simulink model "Estimatoare2021b"  (R2022a)
settings: Solver=VariableStepAuto  StartTime=0.0  StopTime=10  RelTol=1e-3
values from neighbouring files (symbols this model uses):
  AEmd = double(eye(12)+Ts*AE)    [EstimareIntrareNecunoscuta.m]    (also in decuplare.m = double(eye(9)+Ts*Adecup))
  Am = double(round(A(1:9,1:9),4))    [ControllerAroundPointOfOperation.m]    (also in InitializeAircraftPlacePolesCalculateN.m = double(round(A(1:9,1:9),2)); newSys.m)
  Amd = (eye(9)+Ts*Am)    [ControlMinimal.m]    (also in ExtendedControl.m; maimultepuncte.m; newSys.m)
  BEmd = double(Ts*BE)    [EstimareIntrareNecunoscuta.m]    (also in decuplare.m = double(Ts*Bdecup))
  Bm = double(round(B(1:9,1:5),4))    [ControllerAroundPointOfOperation.m]    (also in InitializeAircraftPlacePolesCalculateN.m = double(round(B(1:9,1:5),2)); newSys.m)
  Bmd = Ts*Bm    [ControlMinimal.m]    (also in ExtendedControl.m; maimultepuncte.m; newSys.m)
  CEmd = CE    [EstimareIntrareNecunoscuta.m]    (also in decuplare.m)
  Cm = eye(9)    [newSys.m]
  Cmd = Cm    [ControlMinimal.m]    (also in ExtendedControl.m; maimultepuncte.m; newSys.m)
  F = Ft+Rearth2body(0,Theta,Psi)*Fa+R*G    [aircraftSystem.m]    (also in decuplare.m = T*Adecup-K1*CE; proofCerinteLabEstim.m = T*A-K1*C)
  H = H/z    [ControlMinimal.m]    (also in H.m = [1,tan(Theta)*sin(Phi),tan(Theta)*cos(Phi); decuplare.m = E*pinv(CE*E); proofCerinteLabEstim.m = E*pinv(C*E))
  K = K1+K2    [decuplare.m]
  Km = place(Am,Bm,P)    [ControllerAroundPointOfOperation.m]    (also in InitializeAircraftPlacePolesCalculateN.m; newSys.m)
  Kmd = dlqr(Amd,Bmd,Q,R)    [ControlMinimal.m]    (also in ExtendedControl.m; maimultepuncte.m; newSys.m = lqr(Am-Ld*Cmd,Bm,Q,R))
  L = place(Am',Cm',ObsPoles).'    [newSys.m]
  Ld = place(Amd',Cmd',ObsPoles).'    [newSys.m]
  LEd = place(AEmd',CEmd',ObsPoles).'    [EstimareIntrareNecunoscuta.m]
  pointOfEquilibrium = PointOfEquilibrium(operationStates, operatingInputs ,operatingWinds)    [ControllerAroundPointOfOperation.m]    (also in InitializeAircraftPlacePolesCalculateN.m = PointOfEquilibrium([u0;v0;w0;0;0;0;0;Theta0;Psi0;0;0;100].',; TestMergeFinalLoad.m = PointOfEquilibrium(states,inputs,[-1,-1,-1]); extindere_stari_cu_perturbatie.m = PointOfEquilibrium([u0;0;w0;0;0;0;0;Theta0;Psi0;0;0;100].', ; maimultepuncte.m = GetEquilibriumPoint(UW(i),VW(j),WW(k)))
  T = xinputs(1)    [AMatrixAprox.m]    (also in aircraftSystem.m = u(1); decuplare.m = eye(9)-H*CE; proofCerinteLabEstim.m = eye(3)-H*C)
  Ts = 0.1    [ControlMinimal.m]    (also in EstimareIntrareNecunoscuta.m; ExtendedControl.m; KalmanFilterForExtendedLinearSystem.m; LoadmUltiplePoint.m)
  vant = [1,1,1]*0    [EstimareIntrareNecunoscuta.m]    (also in decuplare.m)
undefined symbols (not defined in the file or in its folder): QExt, RExt
libraries: simulink_extras x7
(part 1 of 2)
settings Model: Creator=Bogdan  LastModifiedBy=Bogdan

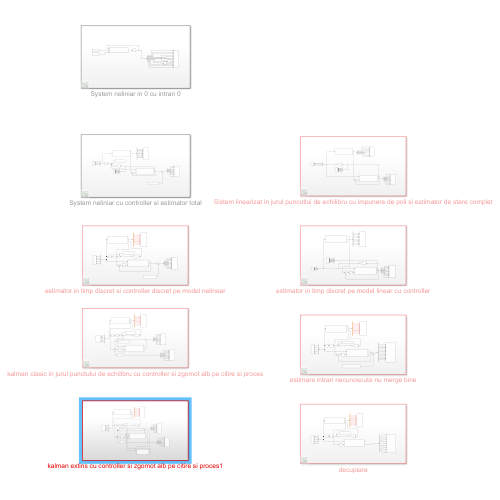
[thumbnail: Simulink's stored preview of the top-level diagram]
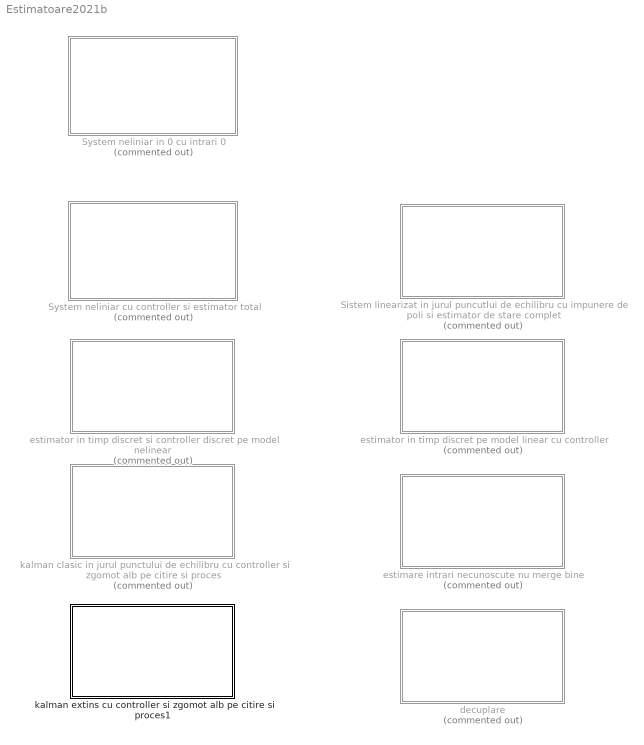
== system Estimatoare2021b ==
  Sistem linearizat in jurul puncutlui de echilibru cu impunere de poli si estimator de stare complet : Subsystem  Description=|  Commented=on
      | Foloseste matricile Am,Bm si Km calculate dupa linearizare in jurul lui 0 cu 
      | %%
      | Am=double(round(A(1:9,1:9),2));
      | Bm=double(round(B(1:9,1:4),2));
      | rank(ctrb(Am,Bm))
      | vpa(eig(Am),2)
      | P=[-.1,-.2,-.3,-.4,-.7,-.8,-1.4,-.15,-7];
      | Km=place(Am,Bm,P)
      | eig(Am-Bm*Km)
  System neliniar cu controller si estimator total : Subsystem  Commented=on
  System neliniar in 0 cu intrari 0 : Subsystem  Commented=on
  decuplare : Subsystem  Description=|  Commented=on
      | Foloseste matricile Am,Bm si Km calculate dupa linearizare in jurul lui 0 cu 
      | %%
      | Am=double(round(A(1:9,1:9),2));
      | Bm=double(round(B(1:9,1:4),2));
      | rank(ctrb(Am,Bm))
      | vpa(eig(Am),2)
      | P=[-.1,-.2,-.3,-.4,-.7,-.8,-1.4,-.15,-7];
      | Km=place(Am,Bm,P)
      | eig(Am-Bm*Km)
  estimare intrari necunoscute nu merge bine : Subsystem  Description=|  Commented=on
      | Foloseste matricile Am,Bm si Km calculate dupa linearizare in jurul lui 0 cu 
      | %%
      | Am=double(round(A(1:9,1:9),2));
      | Bm=double(round(B(1:9,1:4),2));
      | rank(ctrb(Am,Bm))
      | vpa(eig(Am),2)
      | P=[-.1,-.2,-.3,-.4,-.7,-.8,-1.4,-.15,-7];
      | Km=place(Am,Bm,P)
      | eig(Am-Bm*Km)
  estimator in timp discret pe model linear cu controller : Subsystem  Description=|  Commented=on
      | Foloseste matricile Am,Bm si Km calculate dupa linearizare in jurul lui 0 cu 
      | %%
      | Am=double(round(A(1:9,1:9),2));
      | Bm=double(round(B(1:9,1:4),2));
      | rank(ctrb(Am,Bm))
      | vpa(eig(Am),2)
      | P=[-.1,-.2,-.3,-.4,-.7,-.8,-1.4,-.15,-7];
      | Km=place(Am,Bm,P)
      | eig(Am-Bm*Km)
  estimator in timp discret si controller discret pe model nelinear : Subsystem  Description=|  Commented=on
      | Foloseste matricile Am,Bm si Km calculate dupa linearizare in jurul lui 0 cu 
      | %%
      | Am=double(round(A(1:9,1:9),2));
      | Bm=double(round(B(1:9,1:4),2));
      | rank(ctrb(Am,Bm))
      | vpa(eig(Am),2)
      | P=[-.1,-.2,-.3,-.4,-.7,-.8,-1.4,-.15,-7];
      | Km=place(Am,Bm,P)
      | eig(Am-Bm*Km)
  kalman clasic in jurul punctului de echilibru cu controller si zgomot alb pe citire si proces : Subsystem  Description=|  Commented=on
      | Foloseste matricile Am,Bm si Km calculate dupa linearizare in jurul lui 0 cu 
      | %%
      | Am=double(round(A(1:9,1:9),2));
      | Bm=double(round(B(1:9,1:4),2));
      | rank(ctrb(Am,Bm))
      | vpa(eig(Am),2)
      | P=[-.1,-.2,-.3,-.4,-.7,-.8,-1.4,-.15,-7];
      | Km=place(Am,Bm,P)
      | eig(Am-Bm*Km)
  kalman extins cu controller si zgomot alb pe citire si proces1 : Subsystem  Description=|
      | Foloseste matricile Am,Bm si Km calculate dupa linearizare in jurul lui 0 cu 
      | %%
      | Am=double(round(A(1:9,1:9),2));
      | Bm=double(round(B(1:9,1:4),2));
      | rank(ctrb(Am,Bm))
      | vpa(eig(Am),2)
      | P=[-.1,-.2,-.3,-.4,-.7,-.8,-1.4,-.15,-7];
      | Km=place(Am,Bm,P)
      | eig(Am-Bm*Km)

== system Estimatoare2021b/Sistem linearizat in jurul puncutlui de echilibru cu impunere de poli si estimator de stare complet ==
  Controller commands1 : Scope  NumInputPorts=4
  Demux1 : Demux  Outputs=9
  Demux2 : Demux  Outputs=9
  Demux3 : Demux  Outputs=9
  Demux9 : Demux
  Gain1 : Gain  Gain=-Km  Multiplication=Matrix(K*u) (u vector)
  Sum : Sum  Inputs=|+-
  X estim : Scope  NumInputPorts=9
  X real : Scope  NumInputPorts=9
  stari control : Scope  NumInputPorts=9
  system linearizat : Subsystem
  system linearizat1 : Subsystem
  wires:
  Demux9/4 -> Controller commands1/4
  Demux9/2 -> Controller commands1/2
  system linearizat/1(y) -> Sum/1
  Demux9/3 -> Controller commands1/3
  Demux9/1 -> Controller commands1/1
  Demux1/7 -> stari control/7
  Demux1/1 -> stari control/1
  Demux1/8 -> stari control/8
  Demux1/5 -> stari control/5
  Demux1/2 -> stari control/2
  Demux1/3 -> stari control/3
  Demux1/9 -> stari control/9
  Demux1/4 -> stari control/4
  Demux1/6 -> stari control/6
  Demux2/8 -> X real/8
  Demux2/1 -> X real/1
  Demux2/4 -> X real/4
  Demux2/6 -> X real/6
  Demux2/7 -> X real/7
  Demux2/2 -> X real/2
  Demux2/5 -> X real/5
  Demux2/3 -> X real/3
  Demux2/9 -> X real/9
  system linearizat/2(stari) -> Demux2/1
  system linearizat1/1(y_hat) -> Sum/2
  Gain1/1 -> system linearizat1/1(u), system linearizat/1(In1), Demux9/1
  Demux3/5 -> X estim/5
  Demux3/8 -> X estim/8
  Demux3/3 -> X estim/3
  Demux3/2 -> X estim/2
  Demux3/1 -> X estim/1
  Demux3/7 -> X estim/7
  Demux3/4 -> X estim/4
  Demux3/6 -> X estim/6
  Demux3/9 -> X estim/9
  system linearizat1/2(stari) -> Demux3/1
  Sum/1 -> system linearizat1/2(Dy)
  system linearizat1/3(control_states) -> Demux1/1, Gain1/1

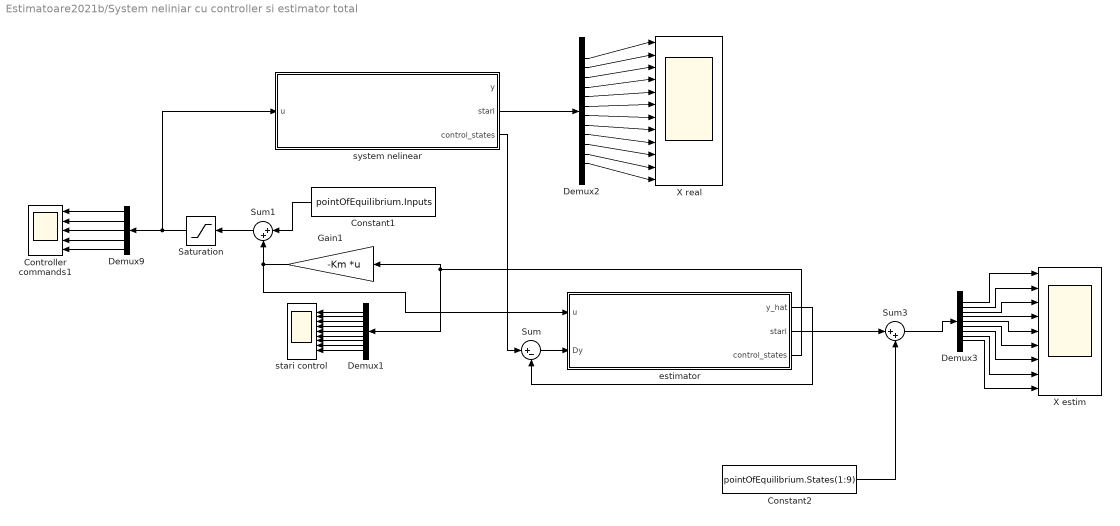
== system Estimatoare2021b/System neliniar cu controller si estimator total ==
  Constant1 : Constant  Value=pointOfEquilibrium.Inputs
  Constant2 : Constant  Value=pointOfEquilibrium.States(1:9)
  Controller commands1 : Scope  NumInputPorts=5
  Demux1 : Demux  Outputs=9
  Demux2 : Demux  Outputs=12
  Demux3 : Demux  Outputs=9
  Demux9 : Demux  Outputs=5
  Gain1 : Gain  Gain=-Km  Multiplication=Matrix(K*u) (u vector)
  Saturation : Saturate  UpperLimit=[10,pi/6,pi/6,pi/6,pi/6]  LowerLimit=[0,-pi/6,-pi/6,-pi/6,-pi/6]
  Sum : Sum  Inputs=|+-
  Sum1 : Sum  Inputs=|++
  Sum3 : Sum  Inputs=|++
  X estim : Scope  NumInputPorts=9
  X real : Scope  NumInputPorts=12
  estimator : Subsystem
  stari control : Scope  NumInputPorts=9
  system nelinear : Subsystem
  wires:
  estimator/1(y_hat) -> Sum/2
  Demux1/8 -> stari control/8
  Demux3/6 -> X estim/6
  system nelinear/2(stari) -> Demux2/1
  Demux3/9 -> X estim/9
  Sum/1 -> estimator/2(Dy)
  Demux1/4 -> stari control/4
  Demux1/3 -> stari control/3
  Demux2/5 -> X real/5
  Demux3/4 -> X estim/4
  Demux2/6 -> X real/6
  Demux2/2 -> X real/2
  Demux3/8 -> X estim/8
  Demux2/9 -> X real/9
  Demux2/8 -> X real/8
  Demux2/3 -> X real/3
  Demux3/2 -> X estim/2
  Demux2/1 -> X real/1
  Demux2/4 -> X real/4
  Demux2/7 -> X real/7
  Demux3/1 -> X estim/1
  Demux3/7 -> X estim/7
  Demux9/1 -> Controller commands1/1
  Demux1/9 -> stari control/9
  Demux1/6 -> stari control/6
  Demux9/3 -> Controller commands1/3
  Demux9/4 -> Controller commands1/4
  Demux1/7 -> stari control/7
  Demux1/2 -> stari control/2
  Demux3/3 -> X estim/3
  Demux1/1 -> stari control/1
  Demux9/2 -> Controller commands1/2
  Demux1/5 -> stari control/5
  Demux3/5 -> X estim/5
  Saturation/1 -> system nelinear/1(u), Demux9/1
  Constant1/1 -> Sum1/1
  Sum1/1 -> Saturation/1
  Gain1/1 -> estimator/1(u), Sum1/2
  estimator/2(stari) -> Sum3/1
  Sum3/1 -> Demux3/1
  Demux2/10 -> X real/10
  Demux2/11 -> X real/11
  Demux2/12 -> X real/12
  Constant2/1 -> Sum3/2
  estimator/3(control_states) -> Gain1/1, Demux1/1
  Demux9/5 -> Controller commands1/5
  system nelinear/3(control_states) -> Sum/1

== system Estimatoare2021b/System neliniar in 0 cu intrari 0 ==
  Constant : Constant  Value=zeros(5,1)
  Constant1 : Constant  Value=zeros(3,1)
  Demux : Demux  Outputs=12
  Integrator : Integrator  InitialCondition=zeros(12,1)
  MATLAB Function : MATLAB Function  TreatAsAtomicUnit=on
  Radians to Degrees : simulink_extras/Transformations/Radians to Degrees
  Radians to Degrees1 : simulink_extras/Transformations/Radians to Degrees
  Radians to Degrees2 : simulink_extras/Transformations/Radians to Degrees
  system states : Scope  NumInputPorts=12
  wires:
  Demux/2 -> system states/2  "v"
  Radians to Degrees2/1 -> system states/9  "Psi"
  Demux/12 -> system states/12  "pozition z in vehicle carried NED"
  MATLAB Function/1(dxdt) -> Integrator/1
  Radians to Degrees/1 -> system states/7  "Phi"
  Demux/10 -> system states/10  "Pozition X in vehicle carried NED"
  Constant/1 -> MATLAB Function/2(u)
  Demux/9 -> Radians to Degrees2/1
  Constant1/1 -> MATLAB Function/3(d)
  Demux/4 -> system states/4  "p"
  Radians to Degrees1/1 -> system states/8  "Theta"
  Demux/3 -> system states/3  "w"
  Integrator/1 -> MATLAB Function/1(x), Demux/1
  Demux/1 -> system states/1  "u"
  Demux/6 -> system states/6  "r"
  Demux/7 -> Radians to Degrees/1
  Demux/8 -> Radians to Degrees1/1
  Demux/11 -> system states/11  "pozition y in vehicle carried NED"
  Demux/5 -> system states/5  "q"

== system Estimatoare2021b/decuplare ==
  Constant1 : Constant  Value=pointOfEquilibrium.Inputs
  Demux : Demux  Outputs=5
  Demux2 : Demux  Outputs=12
  Demux3 : Demux  Outputs=9
  Gain2 : Gain  Gain=-Kmd  Multiplication=Matrix(K*u) (u vector)
  Saturation : Saturate  UpperLimit=[10,pi/6,pi/6,pi/6,pi/6]  LowerLimit=[0,-pi/6,-pi/6,-pi/6,-pi/6]
  Scope : Scope  NumInputPorts=5
  Sum2 : Sum  Inputs=++|
  X estim : Scope  NumInputPorts=9
  X real : Scope  NumInputPorts=12
  Zero-Order Hold : ZeroOrderHold  SampleTime=-1
  Zero-Order Hold1 : ZeroOrderHold  SampleTime=-1
  system linearizat1 : Subsystem
  system nelinear : Subsystem
  wires:
  system nelinear/2(stari) -> Demux2/1
  Demux3/5 -> X estim/5
  Demux3/8 -> X estim/8
  Demux3/3 -> X estim/3
  Demux3/2 -> X estim/2
  Demux3/1 -> X estim/1
  Demux3/7 -> X estim/7
  Demux3/4 -> X estim/4
  Demux3/6 -> X estim/6
  Demux3/9 -> X estim/9
  Demux2/11 -> X real/11
  Demux2/10 -> X real/10
  Demux2/12 -> X real/12
  Demux2/1 -> X real/1
  Demux2/7 -> X real/7
  Demux2/3 -> X real/3
  Demux2/8 -> X real/8
  Demux2/9 -> X real/9
  Demux2/4 -> X real/4
  Demux2/6 -> X real/6
  Demux2/5 -> X real/5
  Demux2/2 -> X real/2
  Gain2/1 -> Sum2/2
  Saturation/1 -> system nelinear/1(u), Demux/1, system linearizat1/1(u)
  Demux/1 -> Scope/1
  Demux/2 -> Scope/2
  Demux/3 -> Scope/3
  Demux/4 -> Scope/4
  Demux/5 -> Scope/5
  Constant1/1 -> Sum2/1
  system nelinear/3(control_states) -> Gain2/1
  system nelinear/1(y) -> Zero-Order Hold/1
  Zero-Order Hold/1 -> system linearizat1/2(Dy)
  Zero-Order Hold1/1 -> Saturation/1
  Sum2/1 -> Zero-Order Hold1/1
  system linearizat1/2(control_states) -> Demux3/1

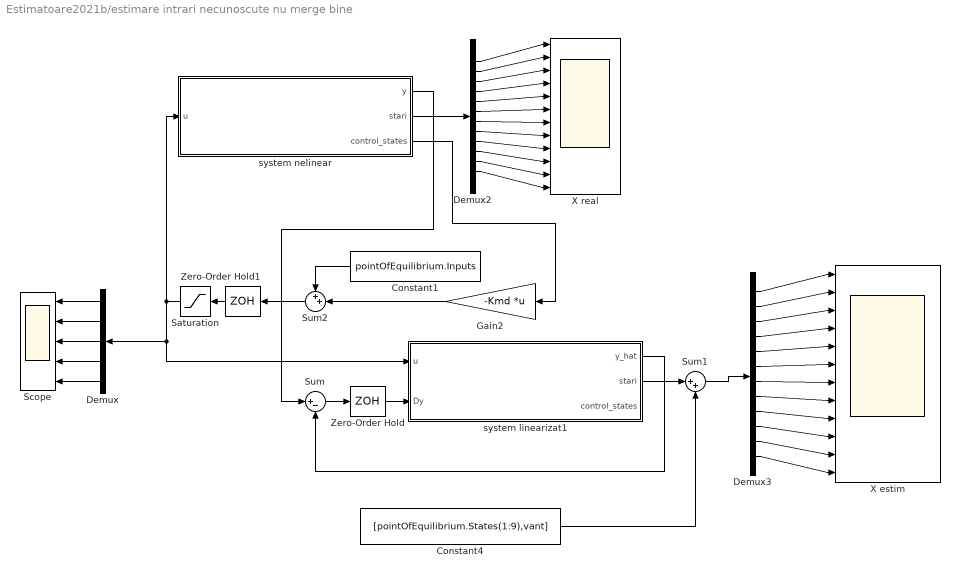
== system Estimatoare2021b/estimare intrari necunoscute nu merge bine ==
  Constant1 : Constant  Value=pointOfEquilibrium.Inputs
  Constant4 : Constant  Value=[pointOfEquilibrium.States(1:9),vant]
  Demux : Demux  Outputs=5
  Demux2 : Demux  Outputs=12
  Demux3 : Demux  Outputs=12
  Gain2 : Gain  Gain=-Kmd  Multiplication=Matrix(K*u) (u vector)
  Saturation : Saturate  UpperLimit=[10,pi/6,pi/6,pi/6,pi/6]  LowerLimit=[0,-pi/6,-pi/6,-pi/6,-pi/6]
  Scope : Scope  NumInputPorts=5
  Sum : Sum  Inputs=|+-
  Sum1 : Sum  Inputs=|++
  Sum2 : Sum  Inputs=++|
  X estim : Scope  NumInputPorts=12
  X real : Scope  NumInputPorts=12
  Zero-Order Hold : ZeroOrderHold  SampleTime=-1
  Zero-Order Hold1 : ZeroOrderHold  SampleTime=-1
  system linearizat1 : Subsystem
  system nelinear : Subsystem
  wires:
  system nelinear/2(stari) -> Demux2/1
  system linearizat1/1(y_hat) -> Sum/2
  Demux3/5 -> X estim/5
  Demux3/8 -> X estim/8
  Demux3/3 -> X estim/3
  Demux3/2 -> X estim/2
  Demux3/1 -> X estim/1
  Demux3/7 -> X estim/7
  Demux3/4 -> X estim/4
  Demux3/6 -> X estim/6
  Demux3/9 -> X estim/9
  Demux2/11 -> X real/11
  Demux2/10 -> X real/10
  Demux2/12 -> X real/12
  Demux2/1 -> X real/1
  Demux2/7 -> X real/7
  Demux2/3 -> X real/3
  Demux2/8 -> X real/8
  Demux2/9 -> X real/9
  Demux2/4 -> X real/4
  Demux2/6 -> X real/6
  Demux2/5 -> X real/5
  Demux2/2 -> X real/2
  Sum1/1 -> Demux3/1
  system linearizat1/2(stari) -> Sum1/1
  Constant4/1 -> Sum1/2
  system nelinear/1(y) -> Sum/1
  Gain2/1 -> Sum2/2
  Saturation/1 -> system nelinear/1(u), Demux/1, system linearizat1/1(u)
  Demux/1 -> Scope/1
  Demux/2 -> Scope/2
  Demux/3 -> Scope/3
  Demux/4 -> Scope/4
  Demux/5 -> Scope/5
  Constant1/1 -> Sum2/1
  Sum/1 -> Zero-Order Hold/1
  Zero-Order Hold/1 -> system linearizat1/2(Dy)
  Zero-Order Hold1/1 -> Saturation/1
  Sum2/1 -> Zero-Order Hold1/1
  Demux3/10 -> X estim/10
  Demux3/11 -> X estim/11
  Demux3/12 -> X estim/12
  system nelinear/3(control_states) -> Gain2/1

== system Estimatoare2021b/estimator in timp discret pe model linear cu controller ==
  Demux : Demux  Outputs=5
  Demux1 : Demux  Outputs=9
  Demux2 : Demux  Outputs=9
  Demux3 : Demux  Outputs=9
  Gain2 : Gain  Gain=-Kmd  Multiplication=Matrix(K*u) (u vector)
  Scope : Scope  NumInputPorts=5
  Sum : Sum  Inputs=|+-
  X estim : Scope  NumInputPorts=9
  X real : Scope  NumInputPorts=9
  Zero-Order Hold2 : ZeroOrderHold  SampleTime=Ts
  stari control : Scope  NumInputPorts=9
  system linearizat : Subsystem
  system linearizat1 : Subsystem
  wires:
  Demux1/7 -> stari control/7
  Demux1/1 -> stari control/1
  Demux1/8 -> stari control/8
  Demux1/5 -> stari control/5
  Demux1/2 -> stari control/2
  Demux1/3 -> stari control/3
  Demux1/9 -> stari control/9
  Demux1/4 -> stari control/4
  Demux1/6 -> stari control/6
  system linearizat/2(stari) -> Demux2/1
  system linearizat1/1(y_hat) -> Sum/2
  Demux3/5 -> X estim/5
  Demux3/8 -> X estim/8
  Demux3/3 -> X estim/3
  Demux3/2 -> X estim/2
  Demux3/1 -> X estim/1
  Demux3/7 -> X estim/7
  Demux3/4 -> X estim/4
  Demux3/6 -> X estim/6
  Demux3/9 -> X estim/9
  system linearizat1/2(stari) -> Demux3/1
  system linearizat/1(y) -> Sum/1
  system linearizat1/3(control_states) -> Gain2/1, Demux1/1
  Gain2/1 -> Demux/1, system linearizat/1(In1), system linearizat1/1(u)
  Zero-Order Hold2/1 -> system linearizat1/2(Dy)
  Sum/1 -> Zero-Order Hold2/1
  Demux2/1 -> X real/1
  Demux2/7 -> X real/7
  Demux2/3 -> X real/3
  Demux2/8 -> X real/8
  Demux2/9 -> X real/9
  Demux2/4 -> X real/4
  Demux2/6 -> X real/6
  Demux2/5 -> X real/5
  Demux2/2 -> X real/2
  Demux/1 -> Scope/1
  Demux/2 -> Scope/2
  Demux/3 -> Scope/3
  Demux/4 -> Scope/4
  Demux/5 -> Scope/5

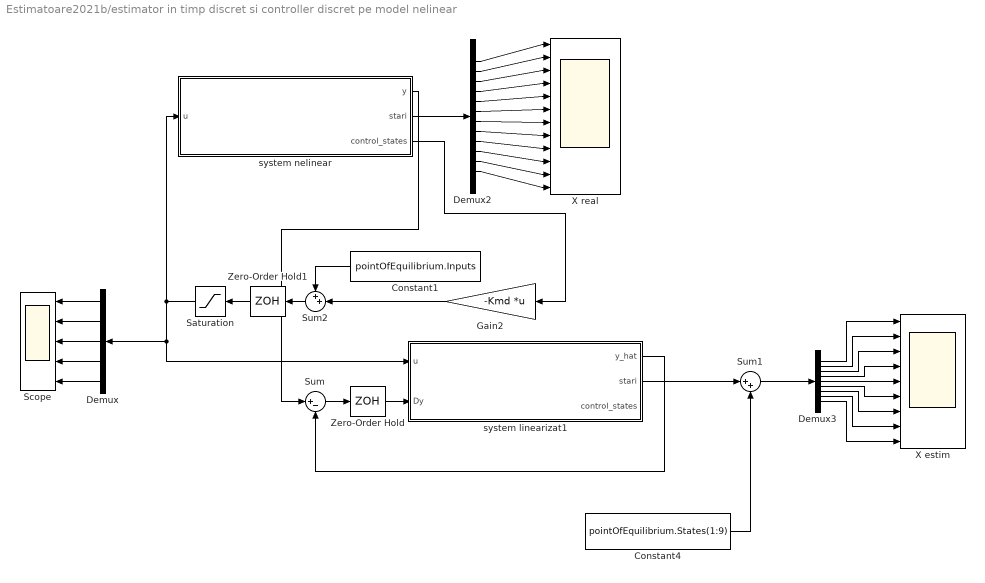
== system Estimatoare2021b/estimator in timp discret si controller discret pe model nelinear ==
  Constant1 : Constant  Value=pointOfEquilibrium.Inputs
  Constant4 : Constant  Value=pointOfEquilibrium.States(1:9)
  Demux : Demux  Outputs=5
  Demux2 : Demux  Outputs=12
  Demux3 : Demux  Outputs=9
  Gain2 : Gain  Gain=-Kmd  Multiplication=Matrix(K*u) (u vector)
  Saturation : Saturate  UpperLimit=[10,pi/6,pi/6,pi/6,pi/6]  LowerLimit=[0,-pi/6,-pi/6,-pi/6,-pi/6]
  Scope : Scope  NumInputPorts=5
  Sum : Sum  Inputs=|+-
  Sum1 : Sum  Inputs=|++
  Sum2 : Sum  Inputs=++|
  X estim : Scope  NumInputPorts=9
  X real : Scope  NumInputPorts=12
  Zero-Order Hold : ZeroOrderHold  SampleTime=-1
  Zero-Order Hold1 : ZeroOrderHold  SampleTime=-1
  system linearizat1 : Subsystem
  system nelinear : Subsystem
  wires:
  system nelinear/2(stari) -> Demux2/1
  system linearizat1/1(y_hat) -> Sum/2
  Demux3/5 -> X estim/5
  Demux3/8 -> X estim/8
  Demux3/3 -> X estim/3
  Demux3/2 -> X estim/2
  Demux3/1 -> X estim/1
  Demux3/7 -> X estim/7
  Demux3/4 -> X estim/4
  Demux3/6 -> X estim/6
  Demux3/9 -> X estim/9
  Demux2/11 -> X real/11
  Demux2/10 -> X real/10
  Demux2/12 -> X real/12
  Demux2/1 -> X real/1
  Demux2/7 -> X real/7
  Demux2/3 -> X real/3
  Demux2/8 -> X real/8
  Demux2/9 -> X real/9
  Demux2/4 -> X real/4
  Demux2/6 -> X real/6
  Demux2/5 -> X real/5
  Demux2/2 -> X real/2
  Sum1/1 -> Demux3/1
  system linearizat1/2(stari) -> Sum1/1
  Constant4/1 -> Sum1/2
  system nelinear/1(y) -> Sum/1
  Gain2/1 -> Sum2/2
  Saturation/1 -> system nelinear/1(u), Demux/1, system linearizat1/1(u)
  Demux/1 -> Scope/1
  Demux/2 -> Scope/2
  Demux/3 -> Scope/3
  Demux/4 -> Scope/4
  Demux/5 -> Scope/5
  Constant1/1 -> Sum2/1
  system nelinear/3(control_states) -> Gain2/1
  Sum/1 -> Zero-Order Hold/1
  Zero-Order Hold/1 -> system linearizat1/2(Dy)
  Zero-Order Hold1/1 -> Saturation/1
  Sum2/1 -> Zero-Order Hold1/1

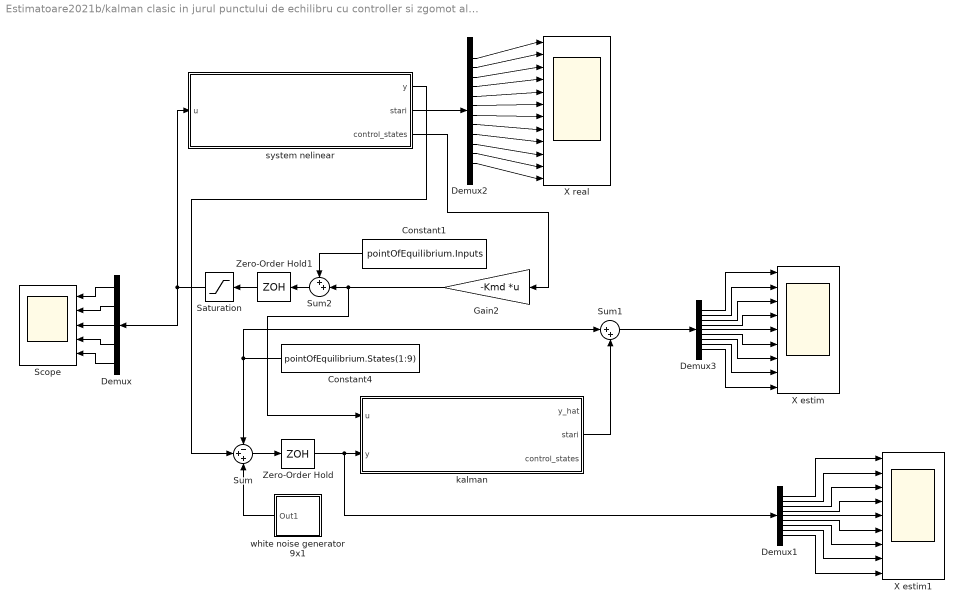
== system Estimatoare2021b/kalman clasic in jurul punctului de echilibru cu controller si zgomot alb pe citire si proces ==
  Constant1 : Constant  Value=pointOfEquilibrium.Inputs
  Constant4 : Constant  Value=pointOfEquilibrium.States(1:9)
  Demux : Demux  Outputs=5
  Demux1 : Demux  Outputs=9
  Demux2 : Demux  Outputs=12
  Demux3 : Demux  Outputs=9
  Gain2 : Gain  Gain=-Kmd  Multiplication=Matrix(K*u) (u vector)
  Saturation : Saturate  UpperLimit=[10,pi/6,pi/6,pi/6,pi/6]  LowerLimit=[0,-pi/6,-pi/6,-pi/6,-pi/6]
  Scope : Scope  NumInputPorts=5
  Sum : Sum  Inputs=-++
  Sum1 : Sum  Inputs=|++
  Sum2 : Sum  Inputs=++|
  X estim : Scope  NumInputPorts=9
  X estim1 : Scope  NumInputPorts=9
  X real : Scope  NumInputPorts=12
  Zero-Order Hold : ZeroOrderHold  SampleTime=-1
  Zero-Order Hold1 : ZeroOrderHold  SampleTime=-1
  kalman : Subsystem
  system nelinear : Subsystem
  white noise generator 9x1 : Subsystem
  wires:
  system nelinear/2(stari) -> Demux2/1
  Demux3/5 -> X estim/5
  Demux3/8 -> X estim/8
  Demux3/3 -> X estim/3
  Demux3/2 -> X estim/2
  Demux3/1 -> X estim/1
  Demux3/7 -> X estim/7
  Demux3/4 -> X estim/4
  Demux3/6 -> X estim/6
  Demux3/9 -> X estim/9
  Demux2/11 -> X real/11
  Demux2/10 -> X real/10
  Demux2/12 -> X real/12
  Demux2/1 -> X real/1
  Demux2/7 -> X real/7
  Demux2/3 -> X real/3
  Demux2/8 -> X real/8
  Demux2/9 -> X real/9
  Demux2/4 -> X real/4
  Demux2/6 -> X real/6
  Demux2/5 -> X real/5
  Demux2/2 -> X real/2
  Gain2/1 -> kalman/1(u), Sum2/2
  Saturation/1 -> system nelinear/1(u), Demux/1
  Demux/1 -> Scope/1
  Demux/2 -> Scope/2
  Demux/3 -> Scope/3
  Demux/4 -> Scope/4
  Demux/5 -> Scope/5
  Constant1/1 -> Sum2/1
  Zero-Order Hold/1 -> Demux1/1, kalman/2(y)
  Zero-Order Hold1/1 -> Saturation/1
  Sum2/1 -> Zero-Order Hold1/1
  Sum/1 -> Zero-Order Hold/1
  Demux1/4 -> X estim1/4
  Demux1/8 -> X estim1/8
  Demux1/7 -> X estim1/7
  Demux1/9 -> X estim1/9
  Demux1/1 -> X estim1/1
  Demux1/6 -> X estim1/6
  Demux1/3 -> X estim1/3
  Demux1/2 -> X estim1/2
  Demux1/5 -> X estim1/5
  white noise generator 9x1/1(Out1) -> Sum/3
  Constant4/1 -> Sum1/1, Sum/1
  system nelinear/1(y) -> Sum/2
  kalman/2(stari) -> Sum1/2
  Sum1/1 -> Demux3/1
  system nelinear/3(control_states) -> Gain2/1

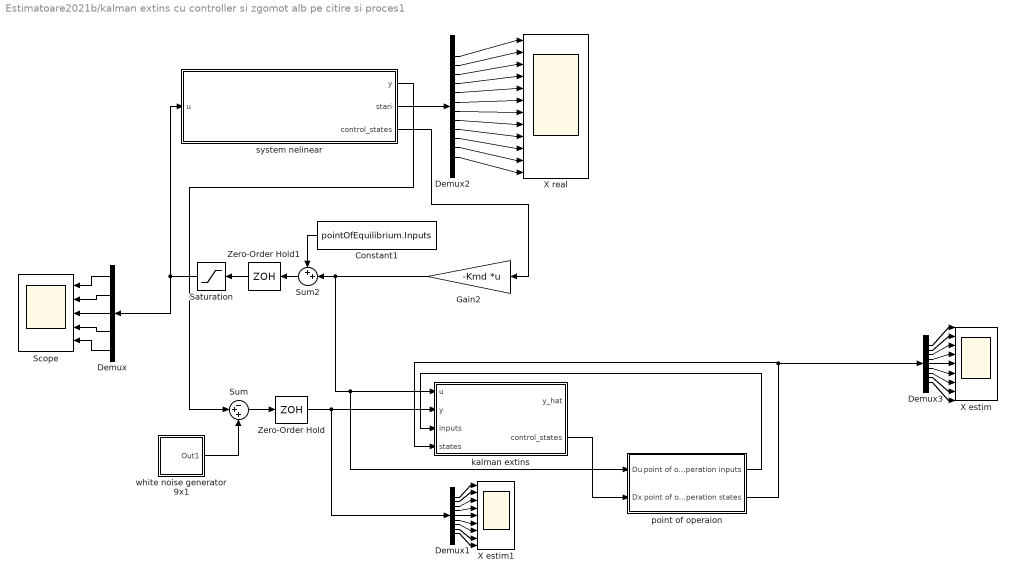
== system Estimatoare2021b/kalman extins cu controller si zgomot alb pe citire si proces1 ==
  Constant1 : Constant  Value=pointOfEquilibrium.Inputs
  Demux : Demux  Outputs=5
  Demux1 : Demux  Outputs=9
  Demux2 : Demux  Outputs=12
  Demux3 : Demux  Outputs=9
  Gain2 : Gain  Gain=-Kmd  Multiplication=Matrix(K*u) (u vector)
  Saturation : Saturate  UpperLimit=[10,pi/6,pi/6,pi/6,pi/6]  LowerLimit=[0,-pi/6,-pi/6,-pi/6,-pi/6]
  Scope : Scope  NumInputPorts=5
  Sum : Sum  Inputs=-++
  Sum2 : Sum  Inputs=++|
  X estim : Scope  NumInputPorts=9
  X estim1 : Scope  NumInputPorts=9
  X real : Scope  NumInputPorts=12
  Zero-Order Hold : ZeroOrderHold  SampleTime=-1
  Zero-Order Hold1 : ZeroOrderHold  SampleTime=-1
  kalman extins : Subsystem
  point of operaion : Subsystem
  system nelinear : Subsystem
  white noise generator 9x1 : Subsystem
  wires:
  system nelinear/2(stari) -> Demux2/1
  Demux3/5 -> X estim/5
  Demux3/8 -> X estim/8
  Demux3/3 -> X estim/3
  Demux3/2 -> X estim/2
  Demux3/1 -> X estim/1
  Demux3/7 -> X estim/7
  Demux3/4 -> X estim/4
  Demux3/6 -> X estim/6
  Demux3/9 -> X estim/9
  Demux2/11 -> X real/11
  Demux2/10 -> X real/10
  Demux2/12 -> X real/12
  Demux2/1 -> X real/1
  Demux2/7 -> X real/7
  Demux2/3 -> X real/3
  Demux2/8 -> X real/8
  Demux2/9 -> X real/9
  Demux2/4 -> X real/4
  Demux2/6 -> X real/6
  Demux2/5 -> X real/5
  Demux2/2 -> X real/2
  Gain2/1 -> point of operaion/1(Du), kalman extins/1(u), Sum2/2
  Saturation/1 -> system nelinear/1(u), Demux/1
  Demux/1 -> Scope/1
  Demux/2 -> Scope/2
  Demux/3 -> Scope/3
  Demux/4 -> Scope/4
  Demux/5 -> Scope/5
  Zero-Order Hold/1 -> Demux1/1, kalman extins/2(y)
  Zero-Order Hold1/1 -> Saturation/1
  Sum2/1 -> Zero-Order Hold1/1
  Sum/1 -> Zero-Order Hold/1
  Demux1/4 -> X estim1/4
  Demux1/8 -> X estim1/8
  Demux1/7 -> X estim1/7
  Demux1/9 -> X estim1/9
  Demux1/1 -> X estim1/1
  Demux1/6 -> X estim1/6
  Demux1/3 -> X estim1/3
  Demux1/2 -> X estim1/2
  Demux1/5 -> X estim1/5
  white noise generator 9x1/1(Out1) -> Sum/3
  system nelinear/1(y) -> Sum/2
  system nelinear/3(control_states) -> Gain2/1
  kalman extins/2(control_states) -> point of operaion/2(Dx)
  Constant1/1 -> Sum2/1
  point of operaion/2(point of operation states) -> Demux3/1, kalman extins/4(states)
  point of operaion/1(point of operation inputs) -> kalman extins/3(inputs)

== system Estimatoare2021b/Sistem linearizat in jurul puncutlui de echilibru cu impunere de poli si estimator de stare complet/system linearizat ==
  In1 : Inport
  Constant1 : Constant  Value=Am
  Constant2 : Constant  Value=Bm
  Constant4 : Constant  Value=pointOfEquilibrium.States(1:9)
  Demux : Demux  Outputs=9
  Gain : Gain  Gain=Cm  Multiplication=Matrix(K*u) (u vector)
  Integrator : Integrator  InitialCondition=pointOfEquilibrium.States(1:9)
  Mux : Mux  Inputs=9
  Product : Product  Multiplication=Matrix(*)
  Product1 : Product  Multiplication=Matrix(*)
  Sum : Sum  Inputs=+++
  Sum1 : Sum  Inputs=+-
  y : Outport
  stari : Outport  Port=2
  control_states : Outport  Port=3
  wires:
  Constant2/1 -> Product1/1
  Integrator/1 -> Sum1/1
  Constant1/1 -> Product/1
  In1/1 -> Product1/2
  Constant4/1 -> Sum1/2
  Sum1/1 -> stari/1, Product/2, Demux/1, Gain/1
  Gain/1 -> y/1
  Demux/2 -> Mux/2
  Demux/5 -> Mux/5
  Demux/3 -> Mux/3
  Demux/6 -> Mux/6
  Mux/1 -> control_states/1
  Demux/4 -> Mux/4
  Demux/1 -> Mux/1
  Product/1 -> Sum/2
  Product1/1 -> Sum/3
  Sum/1 -> Integrator/1
  Demux/7 -> Mux/7
  Demux/8 -> Mux/8
  Demux/9 -> Mux/9

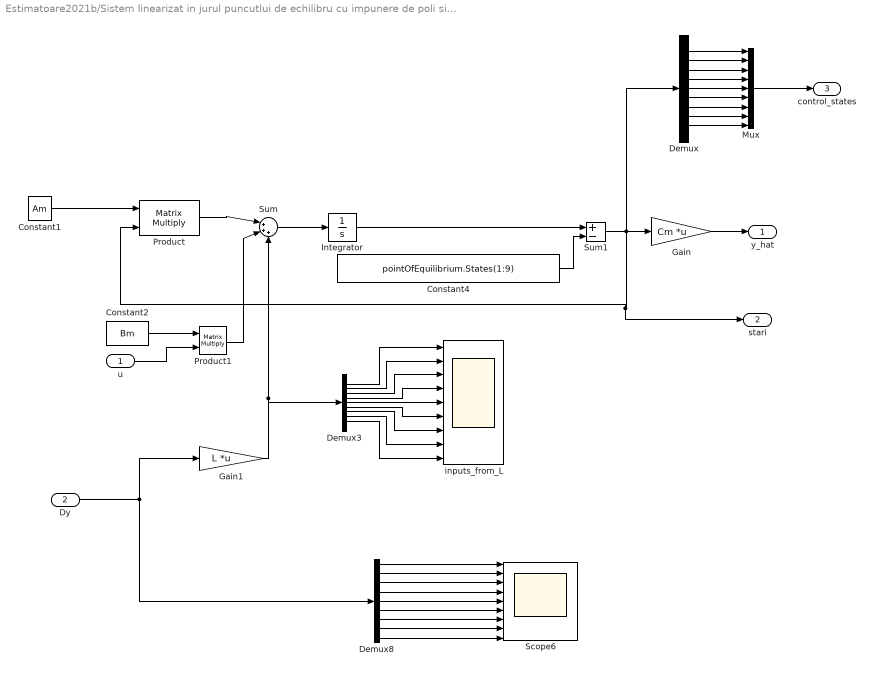
== system Estimatoare2021b/Sistem linearizat in jurul puncutlui de echilibru cu impunere de poli si estimator de stare complet/system linearizat1 ==
  u : Inport
  Dy : Inport  Port=2
  Constant1 : Constant  Value=Am
  Constant2 : Constant  Value=Bm
  Constant4 : Constant  Value=pointOfEquilibrium.States(1:9)
  Demux : Demux  Outputs=9
  Demux3 : Demux  Outputs=9
  Demux8 : Demux  Outputs=9
  Gain : Gain  Gain=Cm  Multiplication=Matrix(K*u) (u vector)
  Gain1 : Gain  Gain=L  Multiplication=Matrix(K*u) (u vector)
  Integrator : Integrator  InitialCondition=pointOfEquilibrium.States(1:9)+error(1:9)
  Mux : Mux  Inputs=9
  Product : Product  Multiplication=Matrix(*)
  Product1 : Product  Multiplication=Matrix(*)
  Scope6 : Scope  NumInputPorts=9
  Sum : Sum  Inputs=|+++
  Sum1 : Sum  Inputs=+-
  inputs_from_L : Scope  NumInputPorts=9
  y_hat : Outport
  stari : Outport  Port=2
  control_states : Outport  Port=3
  wires:
  Constant2/1 -> Product1/1
  Integrator/1 -> Sum1/1
  Product/1 -> Sum/1
  Constant1/1 -> Product/1
  Product1/1 -> Sum/2
  u/1 -> Product1/2
  Constant4/1 -> Sum1/2
  Sum1/1 -> stari/1, Product/2, Demux/1, Gain/1
  Gain/1 -> y_hat/1
  Demux/2 -> Mux/2
  Demux/5 -> Mux/5
  Demux/3 -> Mux/3
  Demux/6 -> Mux/6
  Mux/1 -> control_states/1
  Demux/4 -> Mux/4
  Demux/1 -> Mux/1
  Gain1/1 -> Sum/3, Demux3/1
  Demux/7 -> Mux/7
  Demux/8 -> Mux/8
  Demux/9 -> Mux/9
  Demux8/7 -> Scope6/7
  Demux8/8 -> Scope6/8
  Demux8/4 -> Scope6/4
  Demux8/6 -> Scope6/6
  Demux8/1 -> Scope6/1
  Demux8/5 -> Scope6/5
  Demux8/9 -> Scope6/9
  Demux8/2 -> Scope6/2
  Demux8/3 -> Scope6/3
  Sum/1 -> Integrator/1
  Dy/1 -> Demux8/1, Gain1/1
  Demux3/9 -> inputs_from_L/9
  Demux3/4 -> inputs_from_L/4
  Demux3/6 -> inputs_from_L/6
  Demux3/1 -> inputs_from_L/1
  Demux3/8 -> inputs_from_L/8
  Demux3/3 -> inputs_from_L/3
  Demux3/2 -> inputs_from_L/2
  Demux3/5 -> inputs_from_L/5
  Demux3/7 -> inputs_from_L/7

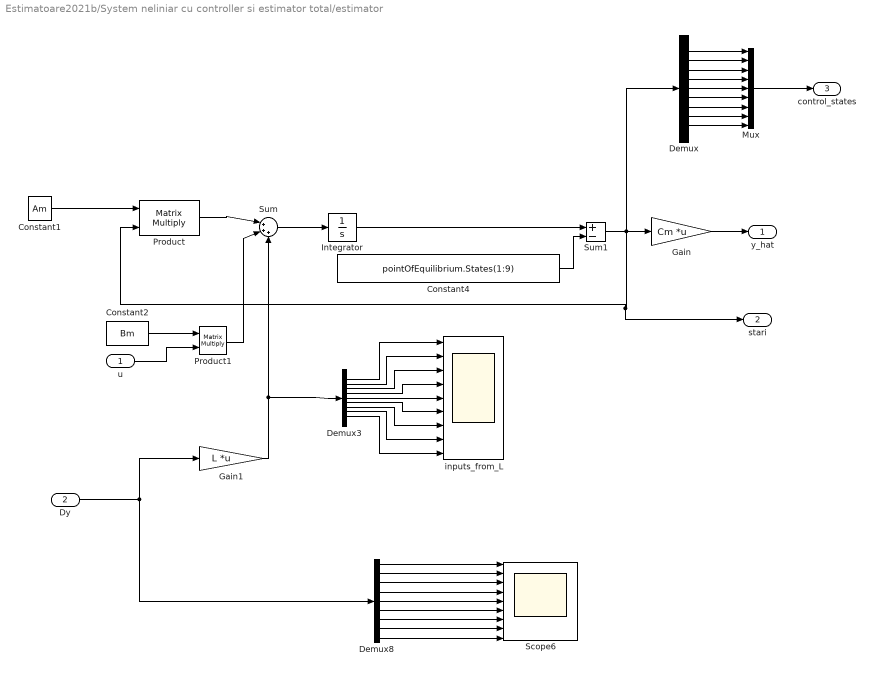
== system Estimatoare2021b/System neliniar cu controller si estimator total/estimator ==
  u : Inport
  Dy : Inport  Port=2
  Constant1 : Constant  Value=Am
  Constant2 : Constant  Value=Bm
  Constant4 : Constant  Value=pointOfEquilibrium.States(1:9)
  Demux : Demux  Outputs=9
  Demux3 : Demux  Outputs=9
  Demux8 : Demux  Outputs=9
  Gain : Gain  Gain=Cm  Multiplication=Matrix(K*u) (u vector)
  Gain1 : Gain  Gain=L  Multiplication=Matrix(K*u) (u vector)
  Integrator : Integrator  InitialCondition=pointOfEquilibrium.States(1:9)+error(1:9)
  Mux : Mux  Inputs=9
  Product : Product  Multiplication=Matrix(*)
  Product1 : Product  Multiplication=Matrix(*)
  Scope6 : Scope  NumInputPorts=9
  Sum : Sum  Inputs=|+++
  Sum1 : Sum  Inputs=+-
  inputs_from_L : Scope  NumInputPorts=9
  y_hat : Outport
  stari : Outport  Port=2
  control_states : Outport  Port=3
  wires:
  Constant2/1 -> Product1/1
  Integrator/1 -> Sum1/1
  Product/1 -> Sum/1
  Constant1/1 -> Product/1
  Product1/1 -> Sum/2
  u/1 -> Product1/2
  Constant4/1 -> Sum1/2
  Sum1/1 -> Demux/1, stari/1, Product/2, Gain/1
  Gain/1 -> y_hat/1
  Demux/2 -> Mux/2
  Demux/5 -> Mux/5
  Demux/3 -> Mux/3
  Demux/6 -> Mux/6
  Mux/1 -> control_states/1
  Demux/4 -> Mux/4
  Demux/1 -> Mux/1
  Gain1/1 -> Sum/3, Demux3/1
  Demux/7 -> Mux/7
  Demux/8 -> Mux/8
  Demux/9 -> Mux/9
  Demux8/7 -> Scope6/7
  Demux8/8 -> Scope6/8
  Demux8/4 -> Scope6/4
  Demux8/6 -> Scope6/6
  Demux8/1 -> Scope6/1
  Demux8/5 -> Scope6/5
  Demux8/9 -> Scope6/9
  Demux8/2 -> Scope6/2
  Demux8/3 -> Scope6/3
  Sum/1 -> Integrator/1
  Dy/1 -> Demux8/1, Gain1/1
  Demux3/9 -> inputs_from_L/9
  Demux3/4 -> inputs_from_L/4
  Demux3/6 -> inputs_from_L/6
  Demux3/1 -> inputs_from_L/1
  Demux3/8 -> inputs_from_L/8
  Demux3/3 -> inputs_from_L/3
  Demux3/2 -> inputs_from_L/2
  Demux3/5 -> inputs_from_L/5
  Demux3/7 -> inputs_from_L/7

== system Estimatoare2021b/System neliniar cu controller si estimator total/system nelinear ==
  u : Inport
  Constant : Constant  Value=zeros(3,1)
  Constant4 : Constant  Value=pointOfEquilibrium.States(1:9)
  Demux : Demux  Outputs=9
  Gain : Gain  Gain=Cm  Multiplication=Matrix(K*u) (u vector)
  Integrator : Integrator  InitialCondition=pointOfEquilibrium.States.'+[.1,.1,.1,0,0,0,0,0,0,10,-35,15].'
  MATLAB Function : MATLAB Function  TreatAsAtomicUnit=on
  Mux : Mux  Inputs=9
  Selector : Selector  InputPortWidth=12  IndexOptions=Index vector (dialog)  Indices=[1:9]  OutputSizes=1
  Sum : Sum  Inputs=|+-
  y : Outport
  stari : Outport  Port=2
  control_states : Outport  Port=3
  wires:
  Gain/1 -> y/1
  Demux/2 -> Mux/2
  Demux/5 -> Mux/5
  Demux/3 -> Mux/3
  Demux/6 -> Mux/6
  Demux/4 -> Mux/4
  Demux/1 -> Mux/1
  Demux/7 -> Mux/7
  Demux/8 -> Mux/8
  Demux/9 -> Mux/9
  MATLAB Function/1(dxdt) -> Integrator/1
  Constant/1 -> MATLAB Function/3(d)
  Integrator/1 -> MATLAB Function/1(x), Selector/1, stari/1
  Selector/1 -> Demux/1, Gain/1
  u/1 -> MATLAB Function/2(u)
  Mux/1 -> Sum/1
  Sum/1 -> control_states/1
  Constant4/1 -> Sum/2

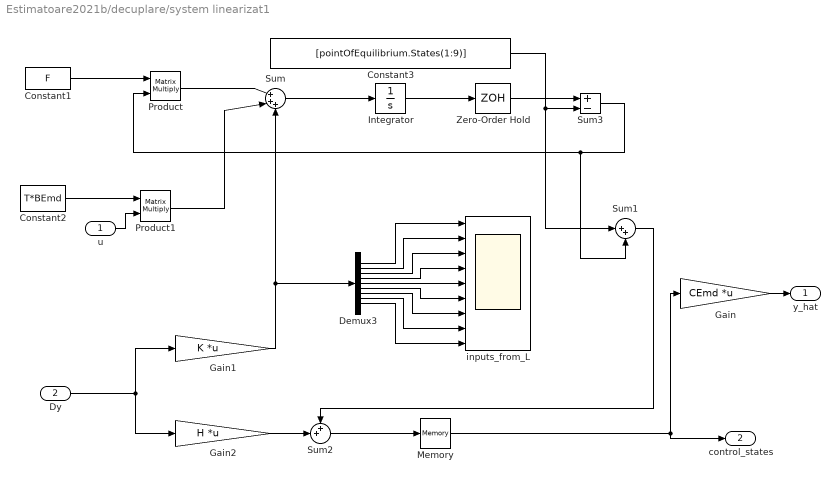
== system Estimatoare2021b/decuplare/system linearizat1 ==
  u : Inport
  Dy : Inport  Port=2
  Constant1 : Constant  Value=F
  Constant2 : Constant  Value=T*BEmd
  Constant3 : Constant  Value=[pointOfEquilibrium.States(1:9)]
  Demux3 : Demux  Outputs=9
  Gain : Gain  Gain=CEmd  Multiplication=Matrix(K*u) (u vector)
  Gain1 : Gain  Gain=K  Multiplication=Matrix(K*u) (u vector)
  Gain2 : Gain  Gain=H  Multiplication=Matrix(K*u) (u vector)
  Integrator : Integrator  InitialCondition=[pointOfEquilibrium.States(1:9)]
  Memory : Memory  InitialCondition=[pointOfEquilibrium.States(1:9)]
  Product : Product  Multiplication=Matrix(*)
  Product1 : Product  Multiplication=Matrix(*)
  Sum : Sum  Inputs=|+++
  Sum1 : Sum  Inputs=|++
  Sum2 : Sum  Inputs=++|
  Sum3 : Sum  Inputs=+-
  Zero-Order Hold : ZeroOrderHold  SampleTime=Ts
  inputs_from_L : Scope  NumInputPorts=9
  y_hat : Outport
  control_states : Outport  Port=2
  wires:
  Constant2/1 -> Product1/1
  Product/1 -> Sum/1
  Constant1/1 -> Product/1
  Product1/1 -> Sum/2
  u/1 -> Product1/2
  Memory/1 -> control_states/1, Gain/1
  Gain1/1 -> Sum/3, Demux3/1
  Sum/1 -> Integrator/1
  Dy/1 -> Gain2/1, Gain1/1
  Demux3/9 -> inputs_from_L/9
  Demux3/4 -> inputs_from_L/4
  Demux3/6 -> inputs_from_L/6
  Demux3/1 -> inputs_from_L/1
  Demux3/8 -> inputs_from_L/8
  Demux3/3 -> inputs_from_L/3
  Demux3/2 -> inputs_from_L/2
  Demux3/5 -> inputs_from_L/5
  Demux3/7 -> inputs_from_L/7
  Integrator/1 -> Zero-Order Hold/1
  Gain/1 -> y_hat/1
  Gain2/1 -> Sum2/2
  Zero-Order Hold/1 -> Sum3/1
  Constant3/1 -> Sum1/1, Sum3/2
  Sum3/1 -> Product/2, Sum1/2
  Sum2/1 -> Memory/1
  Sum1/1 -> Sum2/1

== system Estimatoare2021b/decuplare/system nelinear ==
  u : Inport
  Constant1 : Constant  Value=pointOfEquilibrium.States(1:9)
  Constant4 : Constant  Value=pointOfEquilibrium.States(1:9)
  Demux : Demux  Outputs=9
  Gain : Gain  Gain=Cm  Multiplication=Matrix(K*u) (u vector)
  Integrator : Integrator  InitialCondition=pointOfEquilibrium.States.'+[.2,.1,-.1,0,0,0,0,0,0,10,-35,15].'
  MATLAB Function : MATLAB Function  TreatAsAtomicUnit=on
  Mux : Mux  Inputs=9
  Selector : Selector  InputPortWidth=12  IndexOptions=Index vector (dialog)  Indices=[1:9]  OutputSizes=1
  Sum : Sum  Inputs=|+-
  Sum1 : Sum  Inputs=|+-
  perturbatii : Subsystem
  y : Outport
  stari : Outport  Port=2
  control_states : Outport  Port=3
  wires:
  Gain/1 -> y/1
  Demux/2 -> Mux/2
  Demux/5 -> Mux/5
  Demux/3 -> Mux/3
  Demux/6 -> Mux/6
  Demux/4 -> Mux/4
  Demux/1 -> Mux/1
  Demux/7 -> Mux/7
  Demux/8 -> Mux/8
  Demux/9 -> Mux/9
  MATLAB Function/1(dxdt) -> Integrator/1
  Integrator/1 -> Selector/1, stari/1, MATLAB Function/1(x)
  Selector/1 -> Sum1/1, Demux/1
  u/1 -> MATLAB Function/2(u)
  Mux/1 -> Sum/1
  Sum/1 -> control_states/1
  Constant4/1 -> Sum/2
  perturbatii/1(Out1) -> MATLAB Function/3(d)
  Sum1/1 -> Gain/1
  Constant1/1 -> Sum1/2

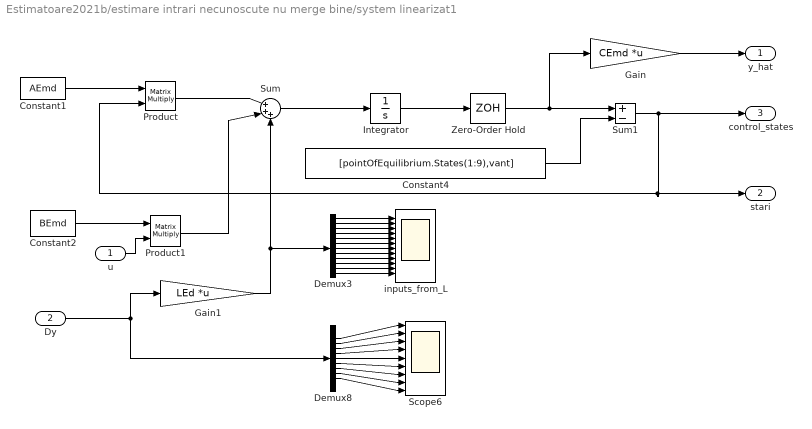
== system Estimatoare2021b/estimare intrari necunoscute nu merge bine/system linearizat1 ==
  u : Inport
  Dy : Inport  Port=2
  Constant1 : Constant  Value=AEmd
  Constant2 : Constant  Value=BEmd
  Constant4 : Constant  Value=[pointOfEquilibrium.States(1:9),vant]
  Demux3 : Demux  Outputs=12
  Demux8 : Demux  Outputs=9
  Gain : Gain  Gain=CEmd  Multiplication=Matrix(K*u) (u vector)
  Gain1 : Gain  Gain=LEd  Multiplication=Matrix(K*u) (u vector)
  Integrator : Integrator  InitialCondition=[pointOfEquilibrium.States(1:9),vant]
  Product : Product  Multiplication=Matrix(*)
  Product1 : Product  Multiplication=Matrix(*)
  Scope6 : Scope  NumInputPorts=9
  Sum : Sum  Inputs=|+++
  Sum1 : Sum  Inputs=+-
  Zero-Order Hold : ZeroOrderHold  SampleTime=Ts
  inputs_from_L : Scope  NumInputPorts=12
  y_hat : Outport
  stari : Outport  Port=2
  control_states : Outport  Port=3
  wires:
  Constant2/1 -> Product1/1
  Product/1 -> Sum/1
  Constant1/1 -> Product/1
  Product1/1 -> Sum/2
  u/1 -> Product1/2
  Constant4/1 -> Sum1/2
  Sum1/1 -> control_states/1, Product/2, stari/1
  Gain1/1 -> Sum/3, Demux3/1
  Demux8/7 -> Scope6/7
  Demux8/8 -> Scope6/8
  Demux8/4 -> Scope6/4
  Demux8/6 -> Scope6/6
  Demux8/1 -> Scope6/1
  Demux8/5 -> Scope6/5
  Demux8/9 -> Scope6/9
  Demux8/2 -> Scope6/2
  Demux8/3 -> Scope6/3
  Sum/1 -> Integrator/1
  Dy/1 -> Demux8/1, Gain1/1
  Demux3/9 -> inputs_from_L/9
  Demux3/4 -> inputs_from_L/4
  Demux3/6 -> inputs_from_L/6
  Demux3/1 -> inputs_from_L/1
  Demux3/8 -> inputs_from_L/8
  Demux3/3 -> inputs_from_L/3
  Demux3/2 -> inputs_from_L/2
  Demux3/5 -> inputs_from_L/5
  Demux3/7 -> inputs_from_L/7
  Integrator/1 -> Zero-Order Hold/1
  Zero-Order Hold/1 -> Gain/1, Sum1/1
  Gain/1 -> y_hat/1
  Demux3/10 -> inputs_from_L/10
  Demux3/11 -> inputs_from_L/11
  Demux3/12 -> inputs_from_L/12

== system Estimatoare2021b/estimare intrari necunoscute nu merge bine/system nelinear ==
  u : Inport
  Constant4 : Constant  Value=pointOfEquilibrium.States(1:9)
  Gain : Gain  Gain=Cm  Multiplication=Matrix(K*u) (u vector)
  Integrator : Integrator  InitialCondition=pointOfEquilibrium.States.'+[0,0,0,0,0,0,0,0,0,10,-35,15].'
  MATLAB Function : MATLAB Function  TreatAsAtomicUnit=on
  Selector : Selector  InputPortWidth=12  IndexOptions=Index vector (dialog)  Indices=[1:9]  OutputSizes=1
  Sum : Sum  Inputs=|+-
  perturbatii : Subsystem
  y : Outport
  stari : Outport  Port=2
  control_states : Outport  Port=3
  wires:
  Gain/1 -> y/1
  MATLAB Function/1(dxdt) -> Integrator/1
  Integrator/1 -> Selector/1, stari/1, MATLAB Function/1(x)
  u/1 -> MATLAB Function/2(u)
  Selector/1 -> Sum/1, Gain/1
  Sum/1 -> control_states/1
  Constant4/1 -> Sum/2
  perturbatii/1(Out1) -> MATLAB Function/3(d)

== system Estimatoare2021b/estimator in timp discret pe model linear cu controller/system linearizat ==
  In1 : Inport
  Constant1 : Constant  Value=Am
  Constant2 : Constant  Value=Bm
  Constant4 : Constant  Value=pointOfEquilibrium.States(1:9)
  Demux : Demux  Outputs=9
  Gain : Gain  Gain=Cm  Multiplication=Matrix(K*u) (u vector)
  Integrator : Integrator  InitialCondition=pointOfEquilibrium.States(1:9)+[.1,.1,.1,0,0,0,0,0,0]
  Mux : Mux  Inputs=9
  Product : Product  Multiplication=Matrix(*)
  Product1 : Product  Multiplication=Matrix(*)
  Sum : Sum  Inputs=+++
  Sum1 : Sum  Inputs=+-
  y : Outport
  stari : Outport  Port=2
  control_states : Outport  Port=3
  wires:
  Constant2/1 -> Product1/1
  Integrator/1 -> Sum1/1
  Constant1/1 -> Product/1
  In1/1 -> Product1/2
  Constant4/1 -> Sum1/2
  Sum1/1 -> stari/1, Product/2, Demux/1, Gain/1
  Gain/1 -> y/1
  Demux/2 -> Mux/2
  Demux/5 -> Mux/5
  Demux/3 -> Mux/3
  Demux/6 -> Mux/6
  Mux/1 -> control_states/1
  Demux/4 -> Mux/4
  Demux/1 -> Mux/1
  Product/1 -> Sum/2
  Product1/1 -> Sum/3
  Sum/1 -> Integrator/1
  Demux/7 -> Mux/7
  Demux/8 -> Mux/8
  Demux/9 -> Mux/9

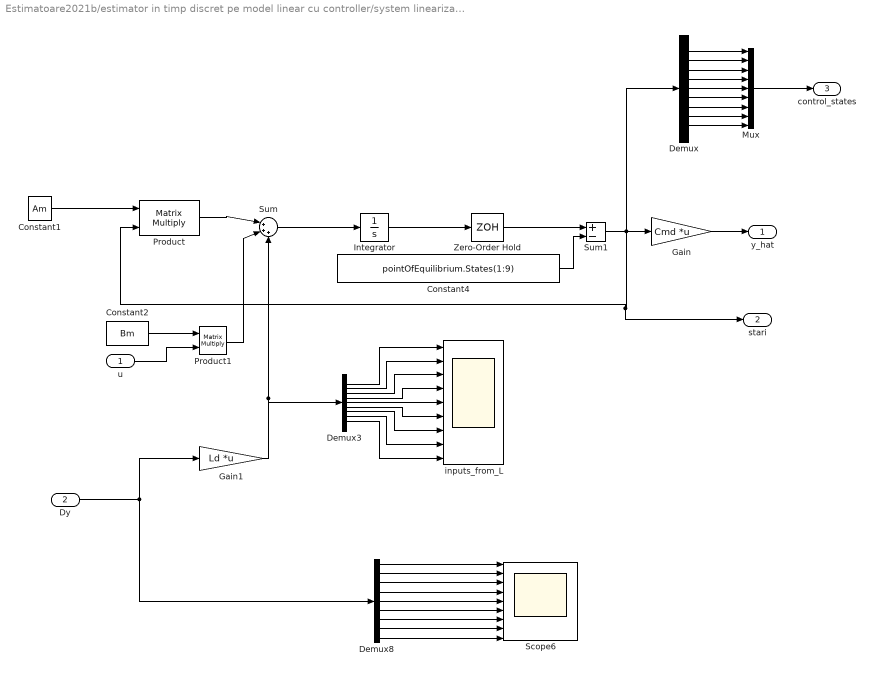
== system Estimatoare2021b/estimator in timp discret pe model linear cu controller/system linearizat1 ==
  u : Inport
  Dy : Inport  Port=2
  Constant1 : Constant  Value=Am
  Constant2 : Constant  Value=Bm
  Constant4 : Constant  Value=pointOfEquilibrium.States(1:9)
  Demux : Demux  Outputs=9
  Demux3 : Demux  Outputs=9
  Demux8 : Demux  Outputs=9
  Gain : Gain  Gain=Cmd  Multiplication=Matrix(K*u) (u vector)
  Gain1 : Gain  Gain=Ld  Multiplication=Matrix(K*u) (u vector)
  Integrator : Integrator  InitialCondition=pointOfEquilibrium.States(1:9)+error(1:9)
  Mux : Mux  Inputs=9
  Product : Product  Multiplication=Matrix(*)
  Product1 : Product  Multiplication=Matrix(*)
  Scope6 : Scope  NumInputPorts=9
  Sum : Sum  Inputs=|+++
  Sum1 : Sum  Inputs=+-
  Zero-Order Hold : ZeroOrderHold  SampleTime=Ts
  inputs_from_L : Scope  NumInputPorts=9
  y_hat : Outport
  stari : Outport  Port=2
  control_states : Outport  Port=3
  wires:
  Constant2/1 -> Product1/1
  Product/1 -> Sum/1
  Constant1/1 -> Product/1
  Product1/1 -> Sum/2
  u/1 -> Product1/2
  Constant4/1 -> Sum1/2
  Sum1/1 -> stari/1, Product/2, Demux/1, Gain/1
  Gain/1 -> y_hat/1
  Demux/2 -> Mux/2
  Demux/5 -> Mux/5
  Demux/3 -> Mux/3
  Demux/6 -> Mux/6
  Mux/1 -> control_states/1
  Demux/4 -> Mux/4
  Demux/1 -> Mux/1
  Gain1/1 -> Sum/3, Demux3/1
  Demux/7 -> Mux/7
  Demux/8 -> Mux/8
  Demux/9 -> Mux/9
  Demux8/7 -> Scope6/7
  Demux8/8 -> Scope6/8
  Demux8/4 -> Scope6/4
  Demux8/6 -> Scope6/6
  Demux8/1 -> Scope6/1
  Demux8/5 -> Scope6/5
  Demux8/9 -> Scope6/9
  Demux8/2 -> Scope6/2
  Demux8/3 -> Scope6/3
  Sum/1 -> Integrator/1
  Dy/1 -> Demux8/1, Gain1/1
  Demux3/9 -> inputs_from_L/9
  Demux3/4 -> inputs_from_L/4
  Demux3/6 -> inputs_from_L/6
  Demux3/1 -> inputs_from_L/1
  Demux3/8 -> inputs_from_L/8
  Demux3/3 -> inputs_from_L/3
  Demux3/2 -> inputs_from_L/2
  Demux3/5 -> inputs_from_L/5
  Demux3/7 -> inputs_from_L/7
  Integrator/1 -> Zero-Order Hold/1
  Zero-Order Hold/1 -> Sum1/1

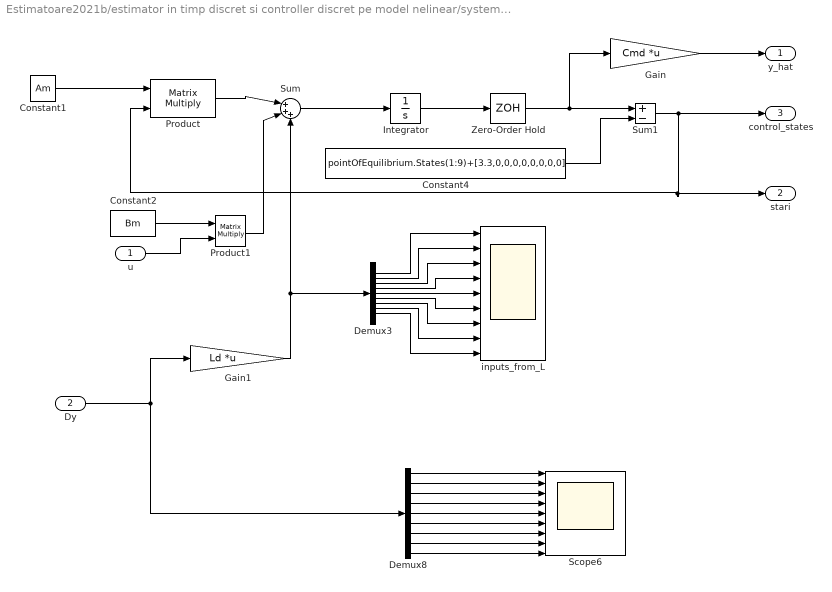
== system Estimatoare2021b/estimator in timp discret si controller discret pe model nelinear/system linearizat1 ==
  u : Inport
  Dy : Inport  Port=2
  Constant1 : Constant  Value=Am
  Constant2 : Constant  Value=Bm
  Constant4 : Constant  Value=pointOfEquilibrium.States(1:9)+[3.3,0,0,0,0,0,0,0,0]
  Demux3 : Demux  Outputs=9
  Demux8 : Demux  Outputs=9
  Gain : Gain  Gain=Cmd  Multiplication=Matrix(K*u) (u vector)
  Gain1 : Gain  Gain=Ld  Multiplication=Matrix(K*u) (u vector)
  Integrator : Integrator  InitialCondition=pointOfEquilibrium.States(1:9)+[3.3,0,0,0,0,0,0,0,0]
  Product : Product  Multiplication=Matrix(*)
  Product1 : Product  Multiplication=Matrix(*)
  Scope6 : Scope  NumInputPorts=9
  Sum : Sum  Inputs=|+++
  Sum1 : Sum  Inputs=+-
  Zero-Order Hold : ZeroOrderHold  SampleTime=Ts
  inputs_from_L : Scope  NumInputPorts=9
  y_hat : Outport
  stari : Outport  Port=2
  control_states : Outport  Port=3
  wires:
  Constant2/1 -> Product1/1
  Product/1 -> Sum/1
  Constant1/1 -> Product/1
  Product1/1 -> Sum/2
  u/1 -> Product1/2
  Constant4/1 -> Sum1/2
  Sum1/1 -> control_states/1, Product/2, stari/1
  Gain1/1 -> Sum/3, Demux3/1
  Demux8/7 -> Scope6/7
  Demux8/8 -> Scope6/8
  Demux8/4 -> Scope6/4
  Demux8/6 -> Scope6/6
  Demux8/1 -> Scope6/1
  Demux8/5 -> Scope6/5
  Demux8/9 -> Scope6/9
  Demux8/2 -> Scope6/2
  Demux8/3 -> Scope6/3
  Sum/1 -> Integrator/1
  Dy/1 -> Demux8/1, Gain1/1
  Demux3/9 -> inputs_from_L/9
  Demux3/4 -> inputs_from_L/4
  Demux3/6 -> inputs_from_L/6
  Demux3/1 -> inputs_from_L/1
  Demux3/8 -> inputs_from_L/8
  Demux3/3 -> inputs_from_L/3
  Demux3/2 -> inputs_from_L/2
  Demux3/5 -> inputs_from_L/5
  Demux3/7 -> inputs_from_L/7
  Integrator/1 -> Zero-Order Hold/1
  Zero-Order Hold/1 -> Gain/1, Sum1/1
  Gain/1 -> y_hat/1

== system Estimatoare2021b/estimator in timp discret si controller discret pe model nelinear/system nelinear ==
  u : Inport
  Constant : Constant  Value=zeros(3,1)
  Constant4 : Constant  Value=pointOfEquilibrium.States(1:9)
  Demux : Demux  Outputs=9
  Gain : Gain  Gain=Cm  Multiplication=Matrix(K*u) (u vector)
  Integrator : Integrator  InitialCondition=pointOfEquilibrium.States.'+[.2,.1,-.1,0,0,0,0,0,0,10,-35,15].'
  MATLAB Function : MATLAB Function  TreatAsAtomicUnit=on
  Mux : Mux  Inputs=9
  Selector : Selector  InputPortWidth=12  IndexOptions=Index vector (dialog)  Indices=[1:9]  OutputSizes=1
  Sum : Sum  Inputs=|+-
  y : Outport
  stari : Outport  Port=2
  control_states : Outport  Port=3
  wires:
  Gain/1 -> y/1
  Demux/2 -> Mux/2
  Demux/5 -> Mux/5
  Demux/3 -> Mux/3
  Demux/6 -> Mux/6
  Demux/4 -> Mux/4
  Demux/1 -> Mux/1
  Demux/7 -> Mux/7
  Demux/8 -> Mux/8
  Demux/9 -> Mux/9
  MATLAB Function/1(dxdt) -> Integrator/1
  Constant/1 -> MATLAB Function/3(d)
  Integrator/1 -> MATLAB Function/1(x), Selector/1, stari/1
  Selector/1 -> Demux/1, Gain/1
  u/1 -> MATLAB Function/2(u)
  Mux/1 -> Sum/1
  Sum/1 -> control_states/1
  Constant4/1 -> Sum/2

== system Estimatoare2021b/kalman clasic in jurul punctului de echilibru cu controller si zgomot alb pe citire si proces/kalman ==
  u : Inport
  y : Inport  Port=2
  Constant : Constant  Value=Cmd
  Constant1 : Constant  Value=Amd
  Constant2 : Constant  Value=Bmd
  Constant3 : Constant  Value=eye(9)
  Constant5 : Constant  Value=eye(9)*1000
  MATLAB Function : MATLAB Function  TreatAsAtomicUnit=on
  Memory : Memory  InitialCondition=zeros(9,1)
  Memory1 : Memory  InitialCondition=eye(9)*1000
  Product2 : Product  Multiplication=Matrix(*)
  Zero-Order Hold1 : ZeroOrderHold  SampleTime=Ts
  Zero-Order Hold2 : ZeroOrderHold  SampleTime=Ts
  y_hat : Outport
  stari : Outport  Port=2
  control_states : Outport  Port=3
  wires:
  Constant/1 -> Product2/1, MATLAB Function/4(Cd)
  Product2/1 -> y_hat/1
  MATLAB Function/1(xest) -> Memory/1
  Memory/1 -> Zero-Order Hold1/1
  Zero-Order Hold1/1 -> control_states/1, stari/1, MATLAB Function/5(xpred), Product2/2
  y/1 -> MATLAB Function/3(y)
  u/1 -> MATLAB Function/6(u)
  Memory1/1 -> Zero-Order Hold2/1
  MATLAB Function/2(P) -> Memory1/1
  Zero-Order Hold2/1 -> MATLAB Function/7("P ")
  Constant1/1 -> MATLAB Function/1(Ad)
  Constant2/1 -> MATLAB Function/2(Bd)
  Constant3/1 -> MATLAB Function/8(Q)
  Constant5/1 -> MATLAB Function/9(R)

== system Estimatoare2021b/kalman clasic in jurul punctului de echilibru cu controller si zgomot alb pe citire si proces/system nelinear ==
  u : Inport
  Constant4 : Constant  Value=pointOfEquilibrium.States(1:9)
  Demux : Demux  Outputs=9
  Gain : Gain  Gain=Cm  Multiplication=Matrix(K*u) (u vector)
  Integrator : Integrator  InitialCondition=pointOfEquilibrium.States.'
  MATLAB Function : MATLAB Function  TreatAsAtomicUnit=on
  Mux : Mux  Inputs=9
  Selector : Selector  InputPortWidth=12  IndexOptions=Index vector (dialog)  Indices=[1:9]  OutputSizes=1
  Sum : Sum  Inputs=|+-
  Zero-Order Hold : ZeroOrderHold  SampleTime=Ts*10
  white noise generator 9x1 : Subsystem
  y : Outport
  stari : Outport  Port=2
  control_states : Outport  Port=3
  wires:
  Gain/1 -> y/1
  Demux/2 -> Mux/2
  Demux/5 -> Mux/5
  Demux/3 -> Mux/3
  Demux/6 -> Mux/6
  Demux/4 -> Mux/4
  Demux/1 -> Mux/1
  Demux/7 -> Mux/7
  Demux/8 -> Mux/8
  Demux/9 -> Mux/9
  Integrator/1 -> MATLAB Function/1(x), Selector/1, stari/1
  Selector/1 -> Demux/1, Gain/1
  u/1 -> MATLAB Function/2(u)
  Mux/1 -> Sum/1
  Sum/1 -> control_states/1
  Constant4/1 -> Sum/2
  MATLAB Function/1(dxdt) -> Integrator/1
  white noise generator 9x1/1(d) -> Zero-Order Hold/1
  Zero-Order Hold/1 -> MATLAB Function/3(d)

== system Estimatoare2021b/kalman clasic in jurul punctului de echilibru cu controller si zgomot alb pe citire si proces/white noise generator 9x1 ==
  Gain : Gain  Gain=1/2
  Mux : Mux  Inputs=9
  Random Number : RandomNumber  Variance=.1  SampleTime=Ts
  Random Number1 : RandomNumber  Variance=.1  SampleTime=Ts
  Random Number2 : RandomNumber  Variance=.1  SampleTime=Ts
  Random Number3 : RandomNumber  Variance=.01  SampleTime=Ts
  Random Number4 : RandomNumber  Variance=.01  SampleTime=Ts
  Random Number5 : RandomNumber  Variance=.01  SampleTime=Ts
  Random Number6 : RandomNumber  Variance=.005  SampleTime=Ts
  Random Number7 : RandomNumber  Variance=.005  SampleTime=Ts
  Random Number8 : RandomNumber  Variance=.005  SampleTime=Ts
  Out1 : Outport
  wires:
  Random Number7/1 -> Mux/8
  Random Number3/1 -> Mux/4
  Random Number4/1 -> Mux/5
  Random Number2/1 -> Mux/3
  Random Number5/1 -> Mux/6
  Random Number8/1 -> Mux/9
  Random Number6/1 -> Mux/7
  Random Number1/1 -> Mux/2
  Random Number/1 -> Mux/1
  Gain/1 -> Out1/1
  Mux/1 -> Gain/1

== system Estimatoare2021b/kalman extins cu controller si zgomot alb pe citire si proces1/kalman extins ==
  u : Inport
  y : Inport  Port=2
  inputs : Inport  Port=3
  states : Inport  Port=4
  Constant : Constant  Value=Cmd
  Product2 : Product  Multiplication=Matrix(*)
  Subsystem : Subsystem
  y_hat : Outport
  control_states : Outport  Port=2
  wires:
  Constant/1 -> Product2/1
  Product2/1 -> y_hat/1
  Subsystem/1(xest) -> control_states/1, Product2/2
  states/1 -> Subsystem/1(states)
  u/1 -> Subsystem/2(u)
  y/1 -> Subsystem/3(y)
  inputs/1 -> Subsystem/4(u1)

== system Estimatoare2021b/kalman extins cu controller si zgomot alb pe citire si proces1/point of operaion ==
  Du : Inport
  Dx : Inport  Port=2
  Memory1 : Memory  InitialCondition=pointOfEquilibrium.States(1:9)  InheritSampleTime=on
  Memory2 : Memory  InitialCondition=pointOfEquilibrium.Inputs  InheritSampleTime=on
  Sum3 : Sum  Inputs=|++
  Sum4 : Sum  Inputs=|++
  Zero-Order Hold : ZeroOrderHold  SampleTime=Ts
  Zero-Order Hold1 : ZeroOrderHold  SampleTime=Ts
  point of operation inputs : Outport
  point of operation states : Outport  Port=2
  wires:
  Memory2/1 -> point of operation inputs/1, Sum4/2
  Du/1 -> Sum4/1
  Memory1/1 -> point of operation states/1, Sum3/2
  Sum3/1 -> Zero-Order Hold/1
  Zero-Order Hold/1 -> Memory1/1
  Sum4/1 -> Zero-Order Hold1/1
  Zero-Order Hold1/1 -> Memory2/1
  Dx/1 -> Sum3/1

== system Estimatoare2021b/kalman extins cu controller si zgomot alb pe citire si proces1/system nelinear ==
  u : Inport
  Constant4 : Constant  Value=pointOfEquilibrium.States(1:9)
  Demux : Demux  Outputs=9
  Gain : Gain  Gain=Cm  Multiplication=Matrix(K*u) (u vector)
  Integrator : Integrator  InitialCondition=pointOfEquilibrium.States.'
  MATLAB Function : MATLAB Function  TreatAsAtomicUnit=on
  Mux : Mux  Inputs=9
  Selector : Selector  InputPortWidth=12  IndexOptions=Index vector (dialog)  Indices=[1:9]  OutputSizes=1
  Sum : Sum  Inputs=|+-
  Zero-Order Hold : ZeroOrderHold  SampleTime=Ts*10
  white noise generator 9x1 : Subsystem
  y : Outport
  stari : Outport  Port=2
  control_states : Outport  Port=3
  wires:
  Gain/1 -> y/1
  Demux/2 -> Mux/2
  Demux/5 -> Mux/5
  Demux/3 -> Mux/3
  Demux/6 -> Mux/6
  Demux/4 -> Mux/4
  Demux/1 -> Mux/1
  Demux/7 -> Mux/7
  Demux/8 -> Mux/8
  Demux/9 -> Mux/9
  Integrator/1 -> Selector/1, stari/1, MATLAB Function/1(x)
  Selector/1 -> Demux/1, Gain/1
  u/1 -> MATLAB Function/2(u)
  Mux/1 -> Sum/1
  Sum/1 -> control_states/1
  Constant4/1 -> Sum/2
  MATLAB Function/1(dxdt) -> Integrator/1
  white noise generator 9x1/1(d) -> Zero-Order Hold/1
  Zero-Order Hold/1 -> MATLAB Function/3(d)

== system Estimatoare2021b/kalman extins cu controller si zgomot alb pe citire si proces1/white noise generator 9x1 ==
  Gain : Gain  Gain=1/2
  Mux : Mux  Inputs=9
  Random Number : RandomNumber  Variance=.1  SampleTime=Ts
  Random Number1 : RandomNumber  Variance=.1  SampleTime=Ts
  Random Number2 : RandomNumber  Variance=.1  SampleTime=Ts
  Random Number3 : RandomNumber  Variance=.01  SampleTime=Ts
  Random Number4 : RandomNumber  Variance=.01  SampleTime=Ts
  Random Number5 : RandomNumber  Variance=.01  SampleTime=Ts
  Random Number6 : RandomNumber  Variance=.005  SampleTime=Ts
  Random Number7 : RandomNumber  Variance=.005  SampleTime=Ts
  Random Number8 : RandomNumber  Variance=.005  SampleTime=Ts
  Out1 : Outport
  wires:
  Random Number7/1 -> Mux/8
  Random Number3/1 -> Mux/4
  Random Number4/1 -> Mux/5
  Random Number2/1 -> Mux/3
  Random Number5/1 -> Mux/6
  Random Number8/1 -> Mux/9
  Random Number6/1 -> Mux/7
  Random Number1/1 -> Mux/2
  Random Number/1 -> Mux/1
  Gain/1 -> Out1/1
  Mux/1 -> Gain/1

== system Estimatoare2021b/decuplare/system nelinear/perturbatii ==
  Mux1 : Mux  Inputs=3
  Step : Step  Time=10  SampleTime=0
  Step1 : Step  Time=50  SampleTime=0
  Step2 : Step  Time=80  SampleTime=0
  Out1 : Outport
  wires:
  Step/1 -> Mux1/1
  Step1/1 -> Mux1/2
  Step2/1 -> Mux1/3
  Mux1/1 -> Out1/1
